simulink model "DYNctl_ver4_etud_obfusc"  (R2014b)
settings: Solver=ode45  StartTime=0.0  StopTime=tfin  FixedStep=0.001  RelTol=1e-09
values from neighbouring files (symbols this model uses):
  ae1 = 1.3463    [MatlabProjet.m]    (also in bancessai_ini.m)
  ae2 = 349.0774    [MatlabProjet.m]    (also in bancessai_ini.m)
  ae3 = 1450.3848    [MatlabProjet.m]    (also in bancessai_ini.m)
  ae4 = 703344.2113    [MatlabProjet.m]    (also in bancessai_ini.m)
  as1 = 0.052961    [MatlabProjet.m]    (also in bancessai_ini.m = -0.22862)
  as2 = 30.5716    [MatlabProjet.m]    (also in bancessai_ini.m = 176.4976)
  as3 = -1152.4168    [MatlabProjet.m]    (also in bancessai_ini.m = -16589.0203)
  as4 = 344545.4587    [MatlabProjet.m]    (also in bancessai_ini.m = 767085.5302)
  b_E1 = 13.029359254409743    (= 13.0293592544)    [MatlabProjet.m]    (also in bancEssaiConstantes.m; bancessai_ini.m; matrices_syms.m)
  g = 9.81    [MatlabProjet.m]    (also in bancEssaiConstantes.m; bancessai_ini.m; matrices_syms.m; trajectoire.m = sqrt(1 + dy.^2))
  Ixy = 0.0011691    [MatlabProjet.m]    (also in bancEssaiConstantes.m = 0.011691; bancessai_ini.m; matrices_syms.m)
  L_bobine = 115/1000    (= 0.115)    [MatlabProjet.m]    (also in bancEssaiConstantes.m; bancessai_ini.m = 115; matrices_syms.m)
  m_ps = m_plaque + m_sphere    (= 0.433)    [MatlabProjet.m]    (also in bancessai_ini.m; matrices_syms.m)
  m_sphere = 0.008    [MatlabProjet.m]    (also in bancessai_ini.m; matrices_syms.m)
  r_ABC = 95.2 / 1000    (= 0.0952)    [MatlabProjet.m]    (also in bancessai_ini.m; matrices_syms.m)
  R_bobine = 3.6    [MatlabProjet.m]    (also in bancEssaiConstantes.m; bancessai_ini.m; matrices_syms.m)
  XA = r_ABC    (= 0.0952)    [MatlabProjet.m]    (also in bancEssaiConstantes.m; bancessai_ini.m; matrices_syms.m)
  XB = -r_ABC*sind(30)    [MatlabProjet.m]    (also in bancEssaiConstantes.m = -rABC*sind(30); bancessai_ini.m; matrices_syms.m)
  XC = XB    [MatlabProjet.m]    (also in bancEssaiConstantes.m = -rABC*sind(30); bancessai_ini.m; matrices_syms.m)
  XD = r_DEF*sind(30)    [MatlabProjet.m]    (also in bancEssaiConstantes.m = +rDEF*sind(30); bancessai_ini.m; matrices_syms.m)
  XE = -r_DEF    (= -0.08)    [MatlabProjet.m]    (also in bancEssaiConstantes.m; bancessai_ini.m; matrices_syms.m)
  XF = XD    [MatlabProjet.m]    (also in bancEssaiConstantes.m = +rDEF*sind(30); bancessai_ini.m; matrices_syms.m)
  YA = 0    [MatlabProjet.m]    (also in bancEssaiConstantes.m; bancessai_ini.m; matrices_syms.m)
  YB = r_ABC*cosd(30)    [MatlabProjet.m]    (also in bancEssaiConstantes.m = +rABC*cosd(30); bancessai_ini.m; matrices_syms.m)
  YC = -YB    [MatlabProjet.m]    (also in bancEssaiConstantes.m = -rABC*cosd(30); bancessai_ini.m; matrices_syms.m)
  YD = r_DEF*cosd(30)    [MatlabProjet.m]    (also in bancEssaiConstantes.m = +rDEF*cosd(30); bancessai_ini.m; matrices_syms.m)
  YE = 0    [MatlabProjet.m]    (also in bancEssaiConstantes.m; bancessai_ini.m; matrices_syms.m)
  YF = -YD    [MatlabProjet.m]    (also in bancEssaiConstantes.m = -rDEF*cosd(30); bancessai_ini.m; matrices_syms.m)
settings Model: Creator=delafontaine  LastModifiedBy=lemg2013
settings SolverCC: AlgebraicLoopSolver=LineSearch
settings DataIOCC: SignalLoggingSaveFormat=ModelDataLogs
settings DebuggingCC: UnderspecifiedInitializationDetection=Classic  MergeDetectMultiDrivingBlocksExec=none  SolverPrmCheckMsg=none  MultiTaskDSMMsg=warning  MultiTaskCondExecSysMsg=none  FrameProcessingCompatibilityMsg=error
settings RTWCC: IncludeERTFirstTime=on

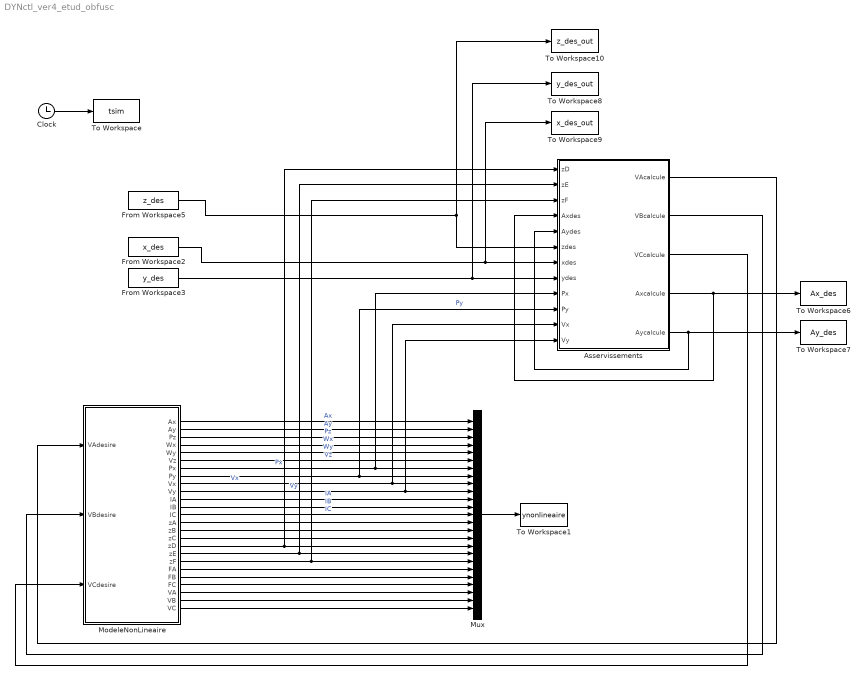
== system DYNctl_ver4_etud_obfusc ==
  Asservissements : Subsystem
      mask help: Simulink:masks:GenSFuncDesc_MD
      mask Help: eval('feval(''rtwprivate'',''rtwhelpview'',''rtw_sfcn_block'')');
  Clock : Clock
  From Workspace2 : FromWorkspace  VariableName=x_des  SampleTime=0  Interpolate=off  OutputAfterFinalValue=Holding final value
  From Workspace3 : FromWorkspace  VariableName=y_des  SampleTime=0  Interpolate=off  OutputAfterFinalValue=Holding final value
  From Workspace5 : FromWorkspace  VariableName=z_des  SampleTime=0  Interpolate=off  OutputAfterFinalValue=Holding final value
  ModeleNonLineaire : Subsystem
      mask help: Simulink:masks:GenSFuncDesc_MD
      mask Help: eval('feval(''rtwprivate'',''rtwhelpview'',''rtw_sfcn_block'')');
  Mux : Mux  Inputs=25
  To Workspace : ToWorkspace  VariableName=tsim  SampleTime=-1
  To Workspace1 : ToWorkspace  VariableName=ynonlineaire  SampleTime=-1
  To Workspace10 : ToWorkspace  VariableName=z_des_out  SampleTime=-1
  To Workspace6 : ToWorkspace  VariableName=Ax_des  SampleTime=-1
  To Workspace7 : ToWorkspace  VariableName=Ay_des  SampleTime=-1
  To Workspace8 : ToWorkspace  VariableName=y_des_out  SampleTime=-1
  To Workspace9 : ToWorkspace  VariableName=x_des_out  SampleTime=-1
  wires:
  Mux/1 -> To Workspace1/1
  Clock/1 -> To Workspace/1
  From Workspace5/1 -> Asservissements/6(zdes), To Workspace10/1
  ModeleNonLineaire/1(Ax) -> Mux/1  "Ax"
  ModeleNonLineaire/2(Ay) -> Mux/2  "Ay"
  ModeleNonLineaire/3(Pz) -> Mux/3  "Pz"
  ModeleNonLineaire/4(Wx) -> Mux/4  "Wx"
  ModeleNonLineaire/5(Wy) -> Mux/5  "Wy"
  ModeleNonLineaire/6(Vz) -> Mux/6  "Vz"
  ModeleNonLineaire/7(Px) -> Asservissements/9(Px), Mux/7  "Px"
  ModeleNonLineaire/8(Py) -> Asservissements/10(Py), Mux/8  "Py"
  ModeleNonLineaire/9(Vx) -> Asservissements/11(Vx), Mux/9  "Vx"
  ModeleNonLineaire/10(Vy) -> Asservissements/12(Vy), Mux/10  "Vy"
  ModeleNonLineaire/11(IA) -> Mux/11  "IA"
  ModeleNonLineaire/12(IB) -> Mux/12  "IB"
  ModeleNonLineaire/13(IC) -> Mux/13  "IC"
  From Workspace3/1 -> Asservissements/8(ydes), To Workspace8/1
  From Workspace2/1 -> Asservissements/7(xdes), To Workspace9/1
  ModeleNonLineaire/20(FA) -> Mux/20
  ModeleNonLineaire/21(FB) -> Mux/21
  ModeleNonLineaire/22(FC) -> Mux/22
  ModeleNonLineaire/23(VA) -> Mux/23
  ModeleNonLineaire/24(VB) -> Mux/24
  ModeleNonLineaire/25(VC) -> Mux/25
  ModeleNonLineaire/17(zD) -> Asservissements/1(zD), Mux/17
  ModeleNonLineaire/18(zE) -> Asservissements/2(zE), Mux/18
  ModeleNonLineaire/19(zF) -> Asservissements/3(zF), Mux/19
  ModeleNonLineaire/14(zA) -> Mux/14
  ModeleNonLineaire/15(zB) -> Mux/15
  ModeleNonLineaire/16(zC) -> Mux/16
  Asservissements/4(Axcalcule) -> Asservissements/4(Axdes), To Workspace6/1
  Asservissements/5(Aycalcule) -> Asservissements/5(Aydes), To Workspace7/1
  Asservissements/1(VAcalcule) -> ModeleNonLineaire/1(VAdesire)
  Asservissements/2(VBcalcule) -> ModeleNonLineaire/2(VBdesire)
  Asservissements/3(VCcalcule) -> ModeleNonLineaire/3(VCdesire)

== system DYNctl_ver4_etud_obfusc/Asservissements ==
  zD : Inport
  zE : Inport  Port=2
  zF : Inport  Port=3
  Axdes : Inport  Port=4
  Aydes : Inport  Port=5
  zdes : Inport  Port=6
  xdes : Inport  Port=7
  ydes : Inport  Port=8
  Px : Inport  Port=9
  Py : Inport  Port=10
  Vx : Inport  Port=11
  Vy : Inport  Port=12
  Asservissements_sfcn : S-Function  FunctionName=Asservissements_sf  SFunctionModules=""  EnableBusSupport=off  mask{rtw_sf_name=Asservissements_sf, showVar=off}
      mask prompts: rtw_sf_name "Simulink:masks:GenSFuncName_MP"; showVar "Simulink:masks:GenSFuncShowModuleList_MP"
      mask help: Simulink:masks:GenSFuncDesc_MD
      mask init:
      | displist = '';
      | if ~strcmp(get_param(gcb, 'FunctionName'), rtw_sf_name);
      |   set_param(gcb, 'FunctionName', rtw_sf_name);
      | end
      | % Check if we are generating code
      | rtw_mode = false;
      | if strcmpi(get_param(bdroot(gcb),'SimulationStatus'),'Initializing')
      | 	rtw_mode = strcmpi(get_param(bdroot(gcb),'BuildingRTWCode'),'on') && ...
      | 		~strcmpi(get_param(bdroot(gcb),'TargetStyle'),'SimulationTarget');
      | end
      | if showVar || rtw_mode
      | 	if exist('rtwsfunc') == 2 | exist('rtwsfunc') == 6
      | 		tmplist = rtwsfunc(rtw_sf_name,gcb);
      | 		tmplist = DAStudio.message('Simulink:masks:GenSFuncListOfModules_IC', tmplist);
      | 	elseif showVar
      | 		tmplist1 = DAStudio.message('Simulink:masks:GenSFuncListOfModules_IC', '');
      |         tmplist2 = DAStudio.message('Simulink:masks:GenSFuncNotLicensed_IC');
      |         tmplist = [tmplist1 tmplist2];
      |  	end
      | end
      | if showVar
      |   displist = tmplist;
      | end
      settings: CopyFcn=|
      | if ~strcmp(get_param(gcb,'Linkstatus'),'none') && ...
      | ~strcmp(get_param(gcb,'Linkstatus'),'implicit')
      |   set_param(gcb,'LinkStatus','none');
      | end
      mask Help: eval('feval(''rtwprivate'',''rtwhelpview'',''rtw_sfcn_block'')');
      mask Display:
      | port_label('input',1,'zD');
      | port_label('input',2,'zE');
      | port_label('input',3,'zF');
      | port_label('input',4,'Axdes');
      | port_label('input',5,'Aydes');
      | port_label('input',6,'zdes');
      | port_label('input',7,'xdes');
      | port_label('input',8,'ydes');
      | port_label('input',9,'Px');
      | port_label('input',10,'Py');
      | port_label('input',11,'Vx');
      | port_label('input',12,'Vy');
      | port_label('output',1,'VAcalcule');
      | port_label('output',2,'VBcalcule');
      | port_label('output',3,'VCcalcule');
      | port_label('output',4,'Axcalcule');
      | port_label('output',5,'Aycalcule');
  __InputSSForSFun__ : Subsystem
  __OutputSSForSFun__ : Subsystem
  VAcalcule : Outport
  VBcalcule : Outport  Port=2
  VCcalcule : Outport  Port=3
  Axcalcule : Outport  Port=4
  Aycalcule : Outport  Port=5
  wires:
  zD/1 -> __InputSSForSFun__/1(zD)
  zE/1 -> __InputSSForSFun__/2(zE)
  zF/1 -> __InputSSForSFun__/3(zF)
  Axdes/1 -> __InputSSForSFun__/4(Axdes)
  Aydes/1 -> __InputSSForSFun__/5(Aydes)
  zdes/1 -> __InputSSForSFun__/6(zdes)
  xdes/1 -> __InputSSForSFun__/7(xdes)
  ydes/1 -> __InputSSForSFun__/8(ydes)
  Px/1 -> __InputSSForSFun__/9(Px)
  Py/1 -> __InputSSForSFun__/10(Py)
  Vx/1 -> __InputSSForSFun__/11(Vx)
  Vy/1 -> __InputSSForSFun__/12(Vy)
  __InputSSForSFun__/1(__UniqueOutportName__1__) -> Asservissements_sfcn/1
  __InputSSForSFun__/2(__UniqueOutportName__2__) -> Asservissements_sfcn/2
  __InputSSForSFun__/3(__UniqueOutportName__3__) -> Asservissements_sfcn/3
  __InputSSForSFun__/4(__UniqueOutportName__4__) -> Asservissements_sfcn/4
  __InputSSForSFun__/5(__UniqueOutportName__5__) -> Asservissements_sfcn/5
  __InputSSForSFun__/6(__UniqueOutportName__6__) -> Asservissements_sfcn/6
  __InputSSForSFun__/7(__UniqueOutportName__7__) -> Asservissements_sfcn/7
  __InputSSForSFun__/8(__UniqueOutportName__8__) -> Asservissements_sfcn/8
  __InputSSForSFun__/9(__UniqueOutportName__9__) -> Asservissements_sfcn/9
  __InputSSForSFun__/10(__UniqueOutportName__10__) -> Asservissements_sfcn/10
  __InputSSForSFun__/11(__UniqueOutportName__11__) -> Asservissements_sfcn/11
  __InputSSForSFun__/12(__UniqueOutportName__12__) -> Asservissements_sfcn/12
  Asservissements_sfcn/1 -> __OutputSSForSFun__/1(__UniqueInportName__1__)
  Asservissements_sfcn/2 -> __OutputSSForSFun__/2(__UniqueInportName__2__)
  Asservissements_sfcn/3 -> __OutputSSForSFun__/3(__UniqueInportName__3__)
  Asservissements_sfcn/4 -> __OutputSSForSFun__/4(__UniqueInportName__4__)
  Asservissements_sfcn/5 -> __OutputSSForSFun__/5(__UniqueInportName__5__)
  __OutputSSForSFun__/1(VAcalcule) -> VAcalcule/1
  __OutputSSForSFun__/2(VBcalcule) -> VBcalcule/1
  __OutputSSForSFun__/3(VCcalcule) -> VCcalcule/1
  __OutputSSForSFun__/4(Axcalcule) -> Axcalcule/1
  __OutputSSForSFun__/5(Aycalcule) -> Aycalcule/1

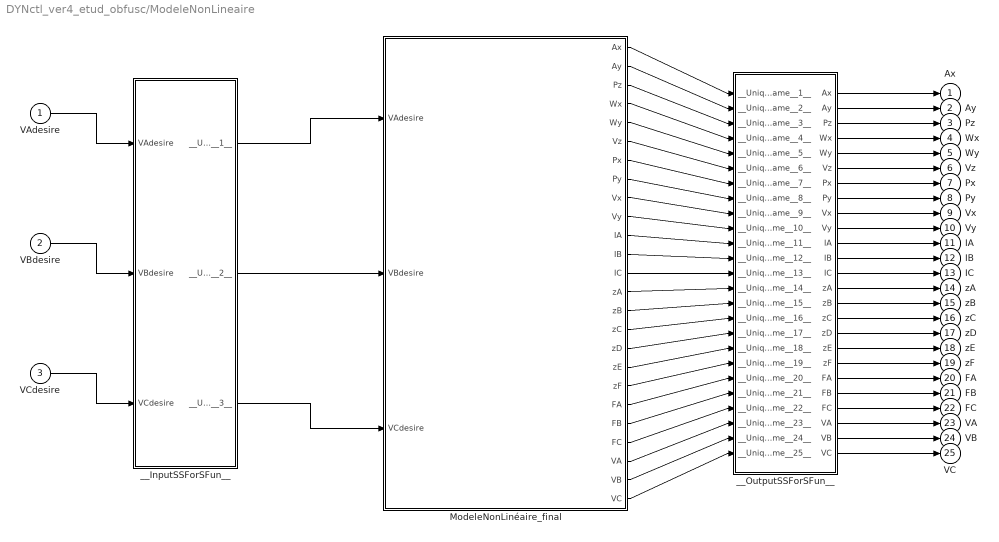
== system DYNctl_ver4_etud_obfusc/ModeleNonLineaire ==
  VAdesire : Inport
  VBdesire : Inport  Port=2
  VCdesire : Inport  Port=3
  ModeleNonLinéaire_final : Subsystem
  __InputSSForSFun__ : Subsystem
  __OutputSSForSFun__ : Subsystem
  Ax : Outport
  Ay : Outport  Port=2
  Pz : Outport  Port=3
  Wx : Outport  Port=4
  Wy : Outport  Port=5
  Vz : Outport  Port=6
  Px : Outport  Port=7
  Py : Outport  Port=8
  Vx : Outport  Port=9
  Vy : Outport  Port=10
  IA : Outport  Port=11
  IB : Outport  Port=12
  IC : Outport  Port=13
  zA : Outport  Port=14
  zB : Outport  Port=15
  zC : Outport  Port=16
  zD : Outport  Port=17
  zE : Outport  Port=18
  zF : Outport  Port=19
  FA : Outport  Port=20
  FB : Outport  Port=21
  FC : Outport  Port=22
  VA : Outport  Port=23
  VB : Outport  Port=24
  VC : Outport  Port=25
  wires:
  VAdesire/1 -> __InputSSForSFun__/1(VAdesire)
  VBdesire/1 -> __InputSSForSFun__/2(VBdesire)
  VCdesire/1 -> __InputSSForSFun__/3(VCdesire)
  __InputSSForSFun__/1(__UniqueOutportName__1__) -> ModeleNonLinéaire_final/1(VAdesire)
  ModeleNonLinéaire_final/1(Ax) -> __OutputSSForSFun__/1(__UniqueInportName__1__)
  ModeleNonLinéaire_final/2(Ay) -> __OutputSSForSFun__/2(__UniqueInportName__2__)
  ModeleNonLinéaire_final/3(Pz) -> __OutputSSForSFun__/3(__UniqueInportName__3__)
  ModeleNonLinéaire_final/4(Wx) -> __OutputSSForSFun__/4(__UniqueInportName__4__)
  ModeleNonLinéaire_final/5(Wy) -> __OutputSSForSFun__/5(__UniqueInportName__5__)
  ModeleNonLinéaire_final/6(Vz) -> __OutputSSForSFun__/6(__UniqueInportName__6__)
  ModeleNonLinéaire_final/7(Px) -> __OutputSSForSFun__/7(__UniqueInportName__7__)
  ModeleNonLinéaire_final/8(Py) -> __OutputSSForSFun__/8(__UniqueInportName__8__)
  ModeleNonLinéaire_final/9(Vx) -> __OutputSSForSFun__/9(__UniqueInportName__9__)
  ModeleNonLinéaire_final/10(Vy) -> __OutputSSForSFun__/10(__UniqueInportName__10__)
  ModeleNonLinéaire_final/11(IA) -> __OutputSSForSFun__/11(__UniqueInportName__11__)
  ModeleNonLinéaire_final/12(IB) -> __OutputSSForSFun__/12(__UniqueInportName__12__)
  ModeleNonLinéaire_final/13(IC) -> __OutputSSForSFun__/13(__UniqueInportName__13__)
  ModeleNonLinéaire_final/14(zA) -> __OutputSSForSFun__/14(__UniqueInportName__14__)
  ModeleNonLinéaire_final/15(zB) -> __OutputSSForSFun__/15(__UniqueInportName__15__)
  ModeleNonLinéaire_final/16(zC) -> __OutputSSForSFun__/16(__UniqueInportName__16__)
  ModeleNonLinéaire_final/17(zD) -> __OutputSSForSFun__/17(__UniqueInportName__17__)
  ModeleNonLinéaire_final/18(zE) -> __OutputSSForSFun__/18(__UniqueInportName__18__)
  ModeleNonLinéaire_final/19(zF) -> __OutputSSForSFun__/19(__UniqueInportName__19__)
  ModeleNonLinéaire_final/20(FA) -> __OutputSSForSFun__/20(__UniqueInportName__20__)
  ModeleNonLinéaire_final/21(FB) -> __OutputSSForSFun__/21(__UniqueInportName__21__)
  ModeleNonLinéaire_final/22(FC) -> __OutputSSForSFun__/22(__UniqueInportName__22__)
  ModeleNonLinéaire_final/23(VA) -> __OutputSSForSFun__/23(__UniqueInportName__23__)
  ModeleNonLinéaire_final/24(VB) -> __OutputSSForSFun__/24(__UniqueInportName__24__)
  ModeleNonLinéaire_final/25(VC) -> __OutputSSForSFun__/25(__UniqueInportName__25__)
  __OutputSSForSFun__/1(Ax) -> Ax/1
  __OutputSSForSFun__/2(Ay) -> Ay/1
  __OutputSSForSFun__/3(Pz) -> Pz/1
  __OutputSSForSFun__/4(Wx) -> Wx/1
  __OutputSSForSFun__/5(Wy) -> Wy/1
  __OutputSSForSFun__/6(Vz) -> Vz/1
  __OutputSSForSFun__/7(Px) -> Px/1
  __OutputSSForSFun__/8(Py) -> Py/1
  __OutputSSForSFun__/9(Vx) -> Vx/1
  __OutputSSForSFun__/10(Vy) -> Vy/1
  __OutputSSForSFun__/11(IA) -> IA/1
  __OutputSSForSFun__/12(IB) -> IB/1
  __OutputSSForSFun__/13(IC) -> IC/1
  __OutputSSForSFun__/14(zA) -> zA/1
  __OutputSSForSFun__/15(zB) -> zB/1
  __OutputSSForSFun__/16(zC) -> zC/1
  __OutputSSForSFun__/17(zD) -> zD/1
  __OutputSSForSFun__/18(zE) -> zE/1
  __OutputSSForSFun__/19(zF) -> zF/1
  __OutputSSForSFun__/20(FA) -> FA/1
  __OutputSSForSFun__/21(FB) -> FB/1
  __OutputSSForSFun__/22(FC) -> FC/1
  __OutputSSForSFun__/23(VA) -> VA/1
  __OutputSSForSFun__/24(VB) -> VB/1
  __OutputSSForSFun__/25(VC) -> VC/1
  __InputSSForSFun__/2(__UniqueOutportName__2__) -> ModeleNonLinéaire_final/2(VBdesire)
  __InputSSForSFun__/3(__UniqueOutportName__3__) -> ModeleNonLinéaire_final/3(VCdesire)

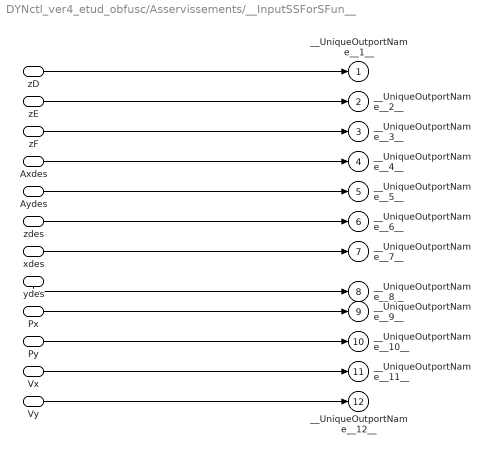
== system DYNctl_ver4_etud_obfusc/Asservissements/__InputSSForSFun__ ==
  zD : Inport
  zE : Inport  Port=2
  zF : Inport  Port=3
  Axdes : Inport  Port=4
  Aydes : Inport  Port=5
  zdes : Inport  Port=6
  xdes : Inport  Port=7
  ydes : Inport  Port=8
  Px : Inport  Port=9
  Py : Inport  Port=10
  Vx : Inport  Port=11
  Vy : Inport  Port=12
  __UniqueOutportName__1__ : Outport
  __UniqueOutportName__2__ : Outport  Port=2
  __UniqueOutportName__3__ : Outport  Port=3
  __UniqueOutportName__4__ : Outport  Port=4
  __UniqueOutportName__5__ : Outport  Port=5
  __UniqueOutportName__6__ : Outport  Port=6
  __UniqueOutportName__7__ : Outport  Port=7
  __UniqueOutportName__8__ : Outport  Port=8
  __UniqueOutportName__9__ : Outport  Port=9
  __UniqueOutportName__10__ : Outport  Port=10
  __UniqueOutportName__11__ : Outport  Port=11
  __UniqueOutportName__12__ : Outport  Port=12
  wires:
  zD/1 -> __UniqueOutportName__1__/1
  zE/1 -> __UniqueOutportName__2__/1
  zF/1 -> __UniqueOutportName__3__/1
  Axdes/1 -> __UniqueOutportName__4__/1
  Aydes/1 -> __UniqueOutportName__5__/1
  zdes/1 -> __UniqueOutportName__6__/1
  xdes/1 -> __UniqueOutportName__7__/1
  ydes/1 -> __UniqueOutportName__8__/1
  Px/1 -> __UniqueOutportName__9__/1
  Py/1 -> __UniqueOutportName__10__/1
  Vx/1 -> __UniqueOutportName__11__/1
  Vy/1 -> __UniqueOutportName__12__/1

== system DYNctl_ver4_etud_obfusc/Asservissements/__OutputSSForSFun__ ==
  __UniqueInportName__1__ : Inport
  __UniqueInportName__2__ : Inport  Port=2
  __UniqueInportName__3__ : Inport  Port=3
  __UniqueInportName__4__ : Inport  Port=4
  __UniqueInportName__5__ : Inport  Port=5
  VAcalcule : Outport
  VBcalcule : Outport  Port=2
  VCcalcule : Outport  Port=3
  Axcalcule : Outport  Port=4
  Aycalcule : Outport  Port=5
  wires:
  __UniqueInportName__1__/1 -> VAcalcule/1
  __UniqueInportName__2__/1 -> VBcalcule/1
  __UniqueInportName__3__/1 -> VCcalcule/1
  __UniqueInportName__4__/1 -> Axcalcule/1  "Ax_des"
  __UniqueInportName__5__/1 -> Aycalcule/1  "Ay_des"

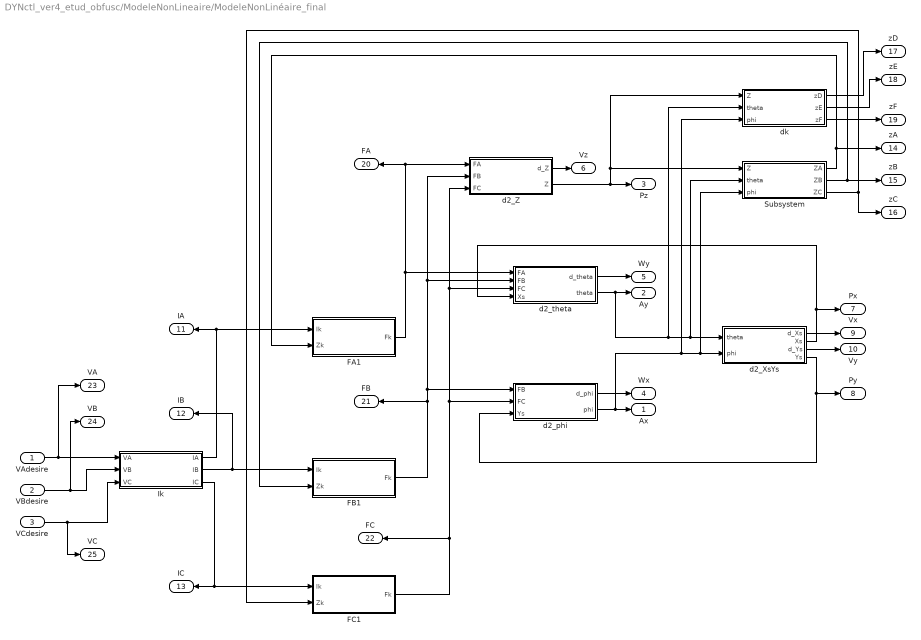
== system DYNctl_ver4_etud_obfusc/ModeleNonLineaire/ModeleNonLinéaire_final ==
  VAdesire : Inport
  VBdesire : Inport  Port=2
  VCdesire : Inport  Port=3
  FA1 : Subsystem
  FB1 : Subsystem
  FC1 : Subsystem
  Ik : Subsystem
  Subsystem : Subsystem
  d2_XsYs : Subsystem
  d2_Z : Subsystem
  d2_phi : Subsystem
  d2_theta : Subsystem
  dk : Subsystem
  Ax : Outport
  Ay : Outport  Port=2
  Pz : Outport  Port=3
  Wx : Outport  Port=4
  Wy : Outport  Port=5
  Vz : Outport  Port=6
  Px : Outport  Port=7
  Py : Outport  Port=8
  Vx : Outport  Port=9
  Vy : Outport  Port=10
  IA : Outport  Port=11
  IB : Outport  Port=12
  IC : Outport  Port=13
  zA : Outport  Port=14
  zB : Outport  Port=15
  zC : Outport  Port=16
  zD : Outport  Port=17
  zE : Outport  Port=18
  zF : Outport  Port=19
  FA : Outport  Port=20
  FB : Outport  Port=21
  FC : Outport  Port=22
  VA : Outport  Port=23
  VB : Outport  Port=24
  VC : Outport  Port=25
  wires:
  VAdesire/1 -> VA/1, Ik/1(VA)
  VBdesire/1 -> VB/1, Ik/2(VB)
  VCdesire/1 -> VC/1, Ik/3(VC)
  Ik/1(IA) -> IA/1, FA1/1(Ik)
  Ik/2(IB) -> IB/1, FB1/1(Ik)
  Ik/3(IC) -> IC/1, FC1/1(Ik)
  FA1/1(Fk) -> d2_theta/1(FA), FA/1, d2_Z/1(FA)
  FB1/1(Fk) -> d2_phi/1(FB), d2_theta/2(FB), d2_Z/2(FB), FB/1
  FC1/1(Fk) -> FC/1, d2_phi/2(FC), d2_theta/3(FC), d2_Z/3(FC)
  d2_phi/2("phi ") -> Ax/1, dk/3(phi), Subsystem/3(phi), d2_XsYs/2(phi)
  d2_theta/2("theta ") -> Ay/1, dk/2(theta), Subsystem/2(theta), d2_XsYs/1(theta)
  d2_XsYs/2(Xs) -> Px/1, d2_theta/4(Xs)
  d2_XsYs/4(Ys) -> Py/1, d2_phi/3(Ys)
  d2_Z/2(Z) -> Pz/1, dk/1(Z), Subsystem/1(Z)
  Subsystem/1(ZA) -> zA/1, FA1/2(Zk)
  Subsystem/2(ZB) -> zB/1, FB1/2(Zk)
  Subsystem/3(ZC) -> zC/1, FC1/2(Zk)
  d2_phi/1("d_phi ") -> Wx/1
  d2_theta/1("d_theta ") -> Wy/1
  d2_Z/1(d_Z) -> Vz/1
  d2_XsYs/1(d_Xs) -> Vx/1
  d2_XsYs/3(d_Ys) -> Vy/1
  dk/1(zD) -> zD/1
  dk/2(zE) -> zE/1
  dk/3(zF) -> zF/1

== system DYNctl_ver4_etud_obfusc/ModeleNonLineaire/__InputSSForSFun__ ==
  VAdesire : Inport
  VBdesire : Inport  Port=2
  VCdesire : Inport  Port=3
  __UniqueOutportName__1__ : Outport
  __UniqueOutportName__2__ : Outport  Port=2
  __UniqueOutportName__3__ : Outport  Port=3
  wires:
  VAdesire/1 -> __UniqueOutportName__1__/1
  VBdesire/1 -> __UniqueOutportName__2__/1
  VCdesire/1 -> __UniqueOutportName__3__/1

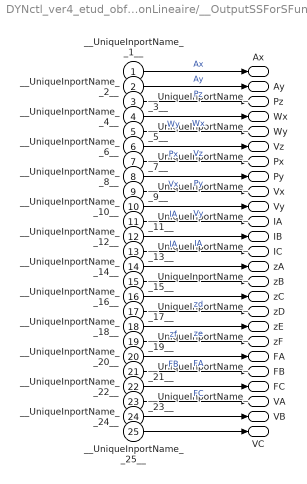
== system DYNctl_ver4_etud_obfusc/ModeleNonLineaire/__OutputSSForSFun__ ==
  __UniqueInportName__1__ : Inport
  __UniqueInportName__2__ : Inport  Port=2
  __UniqueInportName__3__ : Inport  Port=3
  __UniqueInportName__4__ : Inport  Port=4
  __UniqueInportName__5__ : Inport  Port=5
  __UniqueInportName__6__ : Inport  Port=6
  __UniqueInportName__7__ : Inport  Port=7
  __UniqueInportName__8__ : Inport  Port=8
  __UniqueInportName__9__ : Inport  Port=9
  __UniqueInportName__10__ : Inport  Port=10
  __UniqueInportName__11__ : Inport  Port=11
  __UniqueInportName__12__ : Inport  Port=12
  __UniqueInportName__13__ : Inport  Port=13
  __UniqueInportName__14__ : Inport  Port=14
  __UniqueInportName__15__ : Inport  Port=15
  __UniqueInportName__16__ : Inport  Port=16
  __UniqueInportName__17__ : Inport  Port=17
  __UniqueInportName__18__ : Inport  Port=18
  __UniqueInportName__19__ : Inport  Port=19
  __UniqueInportName__20__ : Inport  Port=20
  __UniqueInportName__21__ : Inport  Port=21
  __UniqueInportName__22__ : Inport  Port=22
  __UniqueInportName__23__ : Inport  Port=23
  __UniqueInportName__24__ : Inport  Port=24
  __UniqueInportName__25__ : Inport  Port=25
  Ax : Outport
  Ay : Outport  Port=2
  Pz : Outport  Port=3
  Wx : Outport  Port=4
  Wy : Outport  Port=5
  Vz : Outport  Port=6
  Px : Outport  Port=7
  Py : Outport  Port=8
  Vx : Outport  Port=9
  Vy : Outport  Port=10
  IA : Outport  Port=11
  IB : Outport  Port=12
  IC : Outport  Port=13
  zA : Outport  Port=14
  zB : Outport  Port=15
  zC : Outport  Port=16
  zD : Outport  Port=17
  zE : Outport  Port=18
  zF : Outport  Port=19
  FA : Outport  Port=20
  FB : Outport  Port=21
  FC : Outport  Port=22
  VA : Outport  Port=23
  VB : Outport  Port=24
  VC : Outport  Port=25
  wires:
  __UniqueInportName__1__/1 -> Ax/1  "Ax"
  __UniqueInportName__2__/1 -> Ay/1  "Ay"
  __UniqueInportName__3__/1 -> Pz/1  "Pz"
  __UniqueInportName__4__/1 -> Wx/1  "Wx"
  __UniqueInportName__5__/1 -> Wy/1  "Wy"
  __UniqueInportName__6__/1 -> Vz/1  "Vz"
  __UniqueInportName__7__/1 -> Px/1  "Px"
  __UniqueInportName__8__/1 -> Py/1  "Py"
  __UniqueInportName__9__/1 -> Vx/1  "Vx"
  __UniqueInportName__10__/1 -> Vy/1  "Vy"
  __UniqueInportName__11__/1 -> IA/1  "IA"
  __UniqueInportName__12__/1 -> IB/1  "IA"
  __UniqueInportName__13__/1 -> IC/1  "IA"
  __UniqueInportName__14__/1 -> zA/1
  __UniqueInportName__15__/1 -> zB/1
  __UniqueInportName__16__/1 -> zC/1
  __UniqueInportName__17__/1 -> zD/1  "zd"
  __UniqueInportName__18__/1 -> zE/1  "ze"
  __UniqueInportName__19__/1 -> zF/1  "zf"
  __UniqueInportName__20__/1 -> FA/1  "FA"
  __UniqueInportName__21__/1 -> FB/1  "FB"
  __UniqueInportName__22__/1 -> FC/1  "FC"
  __UniqueInportName__23__/1 -> VA/1
  __UniqueInportName__24__/1 -> VB/1
  __UniqueInportName__25__/1 -> VC/1

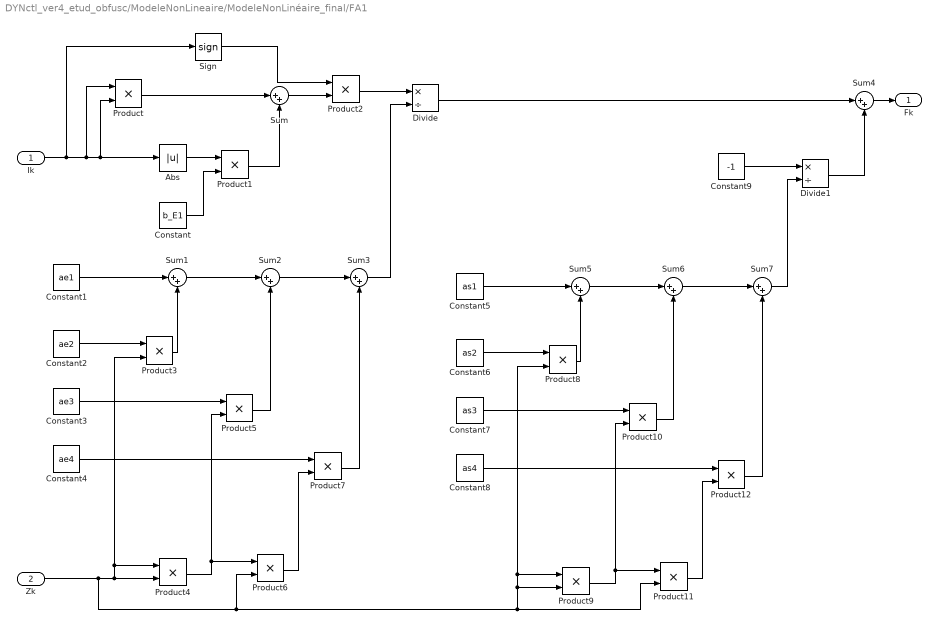
== system DYNctl_ver4_etud_obfusc/ModeleNonLineaire/ModeleNonLinéaire_final/FA1 ==
  Ik : Inport
  Zk : Inport  Port=2
  Abs : Abs
  Constant : Constant  Value=b_E1
  Constant1 : Constant  Value=ae1
  Constant2 : Constant  Value=ae2
  Constant3 : Constant  Value=ae3
  Constant4 : Constant  Value=ae4
  Constant5 : Constant  Value=as1
  Constant6 : Constant  Value=as2
  Constant7 : Constant  Value=as3
  Constant8 : Constant  Value=as4
  Constant9 : Constant  Value=-1
  Divide : Product  Inputs=*/
  Divide1 : Product  Inputs=*/
  Product{,1..12} (13 alike) : Product
  Sign : Signum
  Sum{,1..7} (8 alike) : Sum  Inputs=|++
  Fk : Outport
  wires:
  Ik/1 -> Sign/1, Product/1, Abs/1, Product/2
  Abs/1 -> Product1/1
  Constant/1 -> Product1/2
  Product1/1 -> Sum/2
  Product/1 -> Sum/1
  Sum/1 -> Product2/2
  Sign/1 -> Product2/1
  Constant1/1 -> Sum1/1
  Constant2/1 -> Product3/1
  Product3/1 -> Sum1/2
  Sum1/1 -> Sum2/1
  Product4/1 -> Product6/1, Product5/2
  Constant3/1 -> Product5/1
  Product5/1 -> Sum2/2
  Constant4/1 -> Product7/1
  Product6/1 -> Product7/2
  Product7/1 -> Sum3/2
  Sum2/1 -> Sum3/1
  Product2/1 -> Divide/1
  Sum3/1 -> Divide/2
  Constant5/1 -> Sum5/1
  Constant6/1 -> Product8/1
  Zk/1 -> Product11/2, Product8/2, Product9/1, Product9/2, Product6/2, Product3/2, Product4/1, Product4/2
  Product8/1 -> Sum5/2
  Sum5/1 -> Sum6/1
  Product9/1 -> Product11/1, Product10/2
  Constant7/1 -> Product10/1
  Product10/1 -> Sum6/2
  Constant8/1 -> Product12/1
  Product11/1 -> Product12/2
  Product12/1 -> Sum7/2
  Sum6/1 -> Sum7/1
  Sum7/1 -> Divide1/2
  Divide/1 -> Sum4/1
  Constant9/1 -> Divide1/1
  Divide1/1 -> Sum4/2
  Sum4/1 -> Fk/1

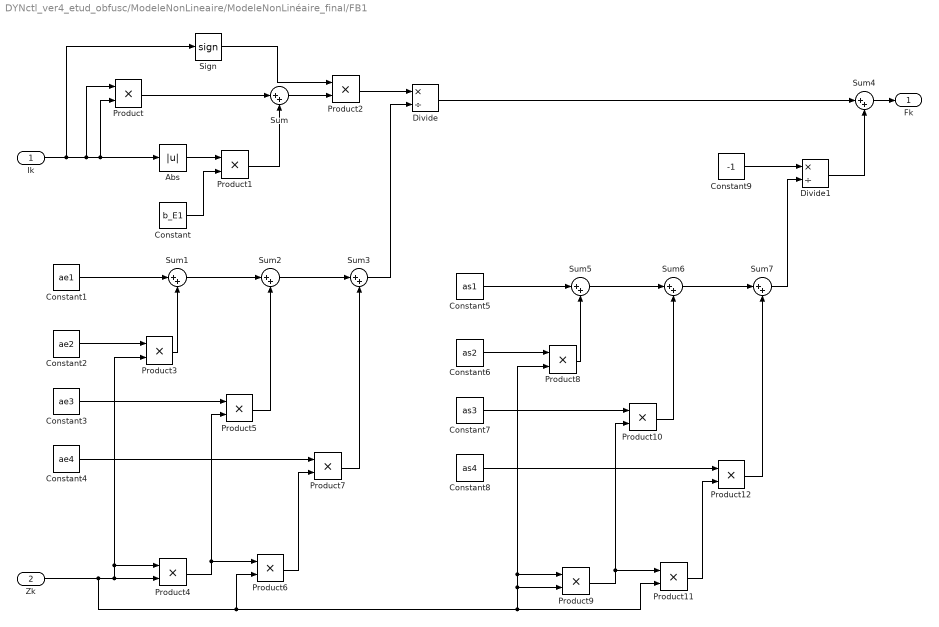
== system DYNctl_ver4_etud_obfusc/ModeleNonLineaire/ModeleNonLinéaire_final/FB1 ==
  Ik : Inport
  Zk : Inport  Port=2
  Abs : Abs
  Constant : Constant  Value=b_E1
  Constant1 : Constant  Value=ae1
  Constant2 : Constant  Value=ae2
  Constant3 : Constant  Value=ae3
  Constant4 : Constant  Value=ae4
  Constant5 : Constant  Value=as1
  Constant6 : Constant  Value=as2
  Constant7 : Constant  Value=as3
  Constant8 : Constant  Value=as4
  Constant9 : Constant  Value=-1
  Divide : Product  Inputs=*/
  Divide1 : Product  Inputs=*/
  Product{,1..12} (13 alike) : Product
  Sign : Signum
  Sum{,1..7} (8 alike) : Sum  Inputs=|++
  Fk : Outport
  wires:
  Ik/1 -> Sign/1, Product/1, Abs/1, Product/2
  Abs/1 -> Product1/1
  Constant/1 -> Product1/2
  Product1/1 -> Sum/2
  Product/1 -> Sum/1
  Sum/1 -> Product2/2
  Sign/1 -> Product2/1
  Constant1/1 -> Sum1/1
  Constant2/1 -> Product3/1
  Product3/1 -> Sum1/2
  Sum1/1 -> Sum2/1
  Product4/1 -> Product6/1, Product5/2
  Constant3/1 -> Product5/1
  Product5/1 -> Sum2/2
  Constant4/1 -> Product7/1
  Product6/1 -> Product7/2
  Product7/1 -> Sum3/2
  Sum2/1 -> Sum3/1
  Product2/1 -> Divide/1
  Sum3/1 -> Divide/2
  Constant5/1 -> Sum5/1
  Constant6/1 -> Product8/1
  Zk/1 -> Product11/2, Product8/2, Product9/1, Product9/2, Product6/2, Product3/2, Product4/1, Product4/2
  Product8/1 -> Sum5/2
  Sum5/1 -> Sum6/1
  Product9/1 -> Product11/1, Product10/2
  Constant7/1 -> Product10/1
  Product10/1 -> Sum6/2
  Constant8/1 -> Product12/1
  Product11/1 -> Product12/2
  Product12/1 -> Sum7/2
  Sum6/1 -> Sum7/1
  Sum7/1 -> Divide1/2
  Divide/1 -> Sum4/1
  Constant9/1 -> Divide1/1
  Divide1/1 -> Sum4/2
  Sum4/1 -> Fk/1

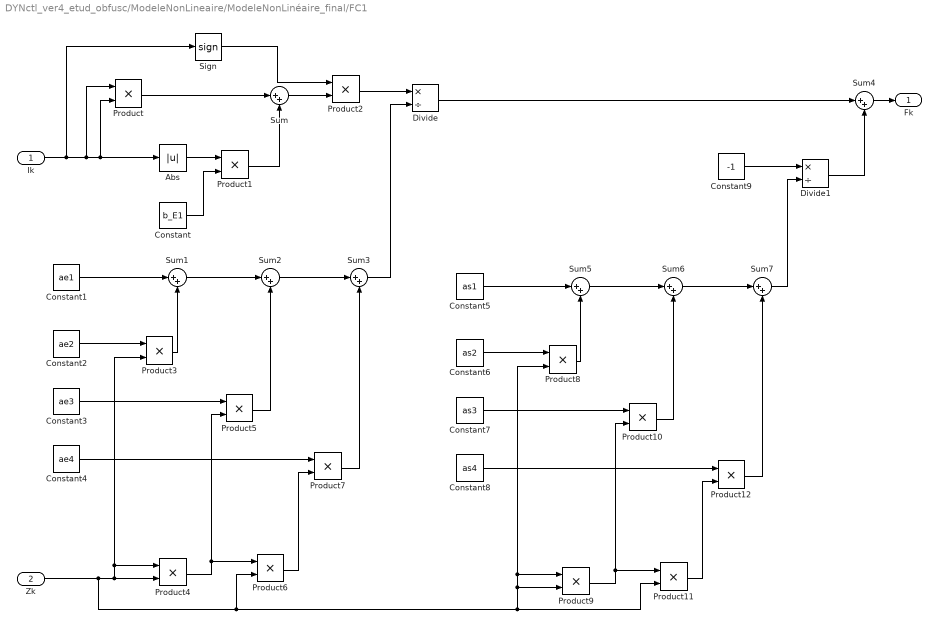
== system DYNctl_ver4_etud_obfusc/ModeleNonLineaire/ModeleNonLinéaire_final/FC1 ==
  Ik : Inport
  Zk : Inport  Port=2
  Abs : Abs
  Constant : Constant  Value=b_E1
  Constant1 : Constant  Value=ae1
  Constant2 : Constant  Value=ae2
  Constant3 : Constant  Value=ae3
  Constant4 : Constant  Value=ae4
  Constant5 : Constant  Value=as1
  Constant6 : Constant  Value=as2
  Constant7 : Constant  Value=as3
  Constant8 : Constant  Value=as4
  Constant9 : Constant  Value=-1
  Divide : Product  Inputs=*/
  Divide1 : Product  Inputs=*/
  Product{,1..12} (13 alike) : Product
  Sign : Signum
  Sum{,1..7} (8 alike) : Sum  Inputs=|++
  Fk : Outport
  wires:
  Ik/1 -> Sign/1, Product/1, Abs/1, Product/2
  Abs/1 -> Product1/1
  Constant/1 -> Product1/2
  Product1/1 -> Sum/2
  Product/1 -> Sum/1
  Sum/1 -> Product2/2
  Sign/1 -> Product2/1
  Constant1/1 -> Sum1/1
  Constant2/1 -> Product3/1
  Product3/1 -> Sum1/2
  Sum1/1 -> Sum2/1
  Product4/1 -> Product6/1, Product5/2
  Constant3/1 -> Product5/1
  Product5/1 -> Sum2/2
  Constant4/1 -> Product7/1
  Product6/1 -> Product7/2
  Product7/1 -> Sum3/2
  Sum2/1 -> Sum3/1
  Product2/1 -> Divide/1
  Sum3/1 -> Divide/2
  Constant5/1 -> Sum5/1
  Constant6/1 -> Product8/1
  Zk/1 -> Product11/2, Product8/2, Product9/1, Product9/2, Product6/2, Product3/2, Product4/1, Product4/2
  Product8/1 -> Sum5/2
  Sum5/1 -> Sum6/1
  Product9/1 -> Product11/1, Product10/2
  Constant7/1 -> Product10/1
  Product10/1 -> Sum6/2
  Constant8/1 -> Product12/1
  Product11/1 -> Product12/2
  Product12/1 -> Sum7/2
  Sum6/1 -> Sum7/1
  Sum7/1 -> Divide1/2
  Divide/1 -> Sum4/1
  Constant9/1 -> Divide1/1
  Divide1/1 -> Sum4/2
  Sum4/1 -> Fk/1

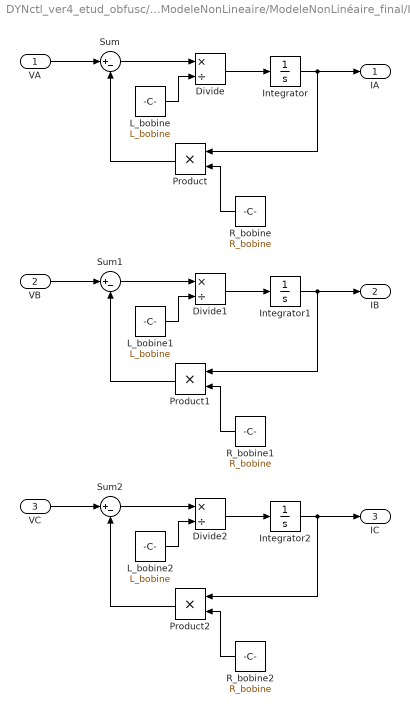
== system DYNctl_ver4_etud_obfusc/ModeleNonLineaire/ModeleNonLinéaire_final/Ik ==
  VA : Inport
  VB : Inport  Port=2
  VC : Inport  Port=3
  Divide : Product  Inputs=*/
  Divide1 : Product  Inputs=*/
  Divide2 : Product  Inputs=*/
  Integrator : Integrator
  Integrator1 : Integrator
  Integrator2 : Integrator
  L_bobine : Constant  Value=L_bobine
  L_bobine1 : Constant  Value=L_bobine
  L_bobine2 : Constant  Value=L_bobine
  Product : Product
  Product1 : Product
  Product2 : Product
  R_bobine : Constant  Value=R_bobine
  R_bobine1 : Constant  Value=R_bobine
  R_bobine2 : Constant  Value=R_bobine
  Sum : Sum  Inputs=|+-
  Sum1 : Sum  Inputs=|+-
  Sum2 : Sum  Inputs=|+-
  IA : Outport
  IB : Outport  Port=2
  IC : Outport  Port=3
  wires:
  Sum/1 -> Divide/1
  L_bobine/1 -> Divide/2
  Divide/1 -> Integrator/1
  Integrator/1 -> IA/1, Product/1
  R_bobine/1 -> Product/2
  Product/1 -> Sum/2
  VA/1 -> Sum/1
  Sum1/1 -> Divide1/1
  L_bobine1/1 -> Divide1/2
  Divide1/1 -> Integrator1/1
  Integrator1/1 -> IB/1, Product1/1
  R_bobine1/1 -> Product1/2
  Product1/1 -> Sum1/2
  VB/1 -> Sum1/1
  Sum2/1 -> Divide2/1
  L_bobine2/1 -> Divide2/2
  Divide2/1 -> Integrator2/1
  Integrator2/1 -> IC/1, Product2/1
  R_bobine2/1 -> Product2/2
  Product2/1 -> Sum2/2
  VC/1 -> Sum2/1

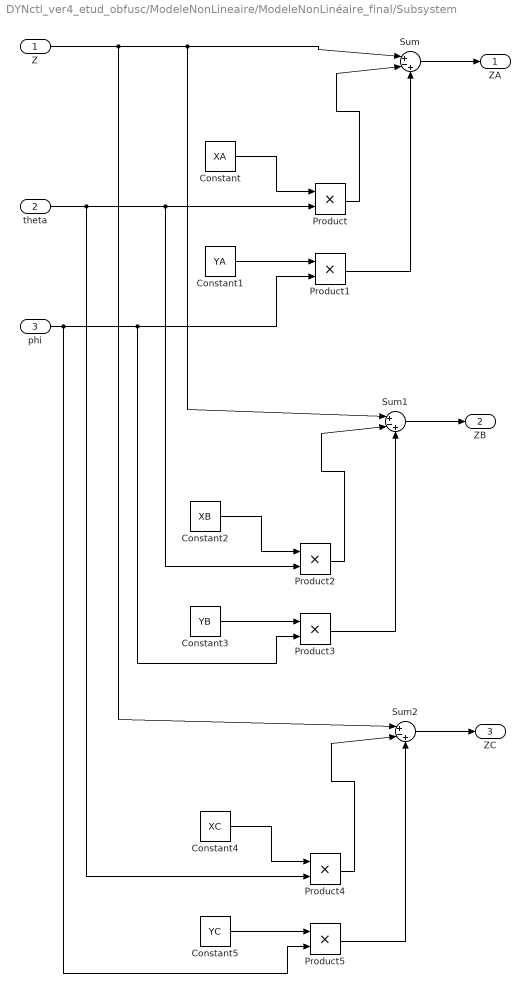
== system DYNctl_ver4_etud_obfusc/ModeleNonLineaire/ModeleNonLinéaire_final/Subsystem ==
  Z : Inport
  theta : Inport  Port=2
  phi : Inport  Port=3
  Constant : Constant  Value=XA
  Constant1 : Constant  Value=YA
  Constant2 : Constant  Value=XB
  Constant3 : Constant  Value=YB
  Constant4 : Constant  Value=XC
  Constant5 : Constant  Value=YC
  Product{,1..5} (6 alike) : Product
  Sum : Sum  Inputs=|+-+
  Sum1 : Sum  Inputs=|+-+
  Sum2 : Sum  Inputs=|+-+
  ZA : Outport
  ZB : Outport  Port=2
  ZC : Outport  Port=3
  wires:
  Constant/1 -> Product/1
  Product/1 -> Sum/2
  Constant1/1 -> Product1/1
  Product1/1 -> Sum/3
  Sum/1 -> ZA/1
  Z/1 -> Sum2/1, Sum1/1, Sum/1
  theta/1 -> Product2/2, Product/2, Product4/2
  Constant2/1 -> Product2/1
  Product2/1 -> Sum1/2
  Constant3/1 -> Product3/1
  phi/1 -> Product3/2, Product1/2, Product5/2
  Product3/1 -> Sum1/3
  Sum1/1 -> ZB/1
  Constant4/1 -> Product4/1
  Product4/1 -> Sum2/2
  Constant5/1 -> Product5/1
  Product5/1 -> Sum2/3
  Sum2/1 -> ZC/1

== system DYNctl_ver4_etud_obfusc/ModeleNonLineaire/ModeleNonLinéaire_final/d2_XsYs ==
  theta : Inport
  phi : Inport  Port=2
  Constant : Constant  Value=-g/1.4
  Constant1 : Constant  Value=g/1.4
  Integrator{,1..3} (4 alike) : Integrator
  Product : Product
  Product1 : Product
  d_Xs : Outport
  Xs : Outport  Port=2
  d_Ys : Outport  Port=3
  Ys : Outport  Port=4
  wires:
  theta/1 -> Product/1
  Constant/1 -> Product/2
  Product/1 -> Integrator/1
  Integrator/1 -> d_Xs/1, Integrator1/1
  Integrator1/1 -> Xs/1
  phi/1 -> Product1/1
  Constant1/1 -> Product1/2
  Product1/1 -> Integrator2/1
  Integrator2/1 -> d_Ys/1, Integrator3/1
  Integrator3/1 -> Ys/1

== system DYNctl_ver4_etud_obfusc/ModeleNonLineaire/ModeleNonLinéaire_final/d2_Z ==
  FA : Inport
  FB : Inport  Port=2
  FC : Inport  Port=3
  Constant : Constant  Value=m_ps
  Constant1 : Constant  Value=g
  Divide : Product  Inputs=*/
  Integrator : Integrator
  Integrator1 : Integrator
  Product : Product
  Sum : Sum  Inputs=++++
  d_Z : Outport
  Z : Outport  Port=2
  wires:
  FB/1 -> Sum/2
  FA/1 -> Sum/1
  FC/1 -> Sum/3
  Constant1/1 -> Product/2
  Product/1 -> Sum/4
  Sum/1 -> Divide/1
  Constant/1 -> Divide/2, Product/1
  Divide/1 -> Integrator/1
  Integrator1/1 -> Z/1
  Integrator/1 -> Integrator1/1, d_Z/1

== system DYNctl_ver4_etud_obfusc/ModeleNonLineaire/ModeleNonLinéaire_final/d2_phi ==
  FB : Inport
  FC : Inport  Port=2
  Ys : Inport  Port=3
  Constant : Constant  Value=Ixy
  Divide : Product  Inputs=*/
  Integrator : Integrator
  Integrator1 : Integrator
  Product{,1..4} (5 alike) : Product
  Sum : Sum  Inputs=|+-
  Sum1 : Sum  Inputs=|++
  cos30 : Constant  Value=cosd(30)
  g : Constant  Value=g
  m_sphere : Constant  Value=m_sphere
  r_ABC : Constant  Value=r_ABC
  "d_phi " : Outport
  "phi " : Outport  Port=2
  wires:
  cos30/1 -> Product/2, Product1/1
  FB/1 -> Product/1
  FC/1 -> Product1/2
  Product/1 -> Sum/1
  Product1/1 -> Sum/2
  Sum/1 -> Product2/1
  r_ABC/1 -> Product2/2
  Product2/1 -> Sum1/1
  m_sphere/1 -> Product3/1
  g/1 -> Product3/2
  Product3/1 -> Product4/2
  Ys/1 -> Product4/1
  Product4/1 -> Sum1/2
  Sum1/1 -> Divide/1
  Constant/1 -> Divide/2
  Divide/1 -> Integrator/1
  Integrator/1 -> "d_phi "/1, Integrator1/1
  Integrator1/1 -> "phi "/1

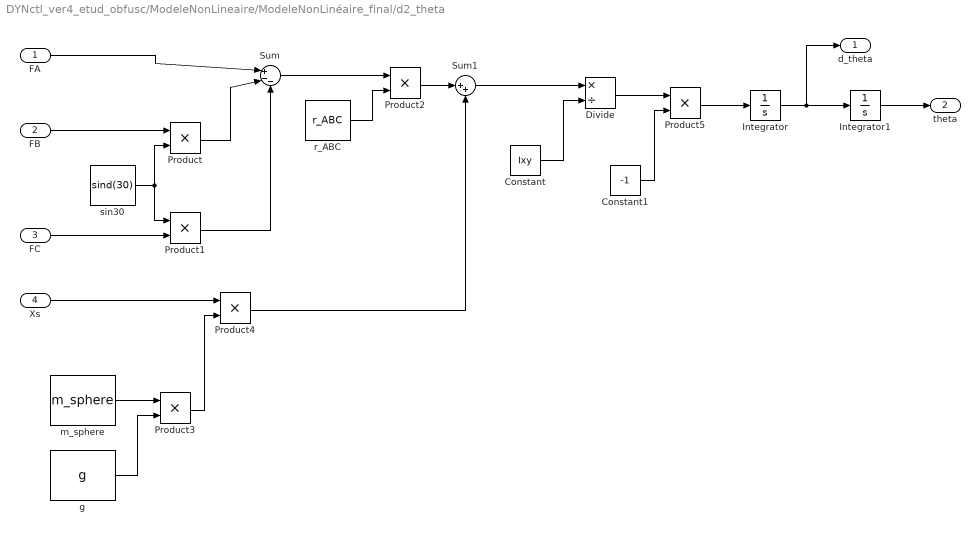
== system DYNctl_ver4_etud_obfusc/ModeleNonLineaire/ModeleNonLinéaire_final/d2_theta ==
  FA : Inport
  FB : Inport  Port=2
  FC : Inport  Port=3
  Xs : Inport  Port=4
  Constant : Constant  Value=Ixy
  Constant1 : Constant  Value=-1
  Divide : Product  Inputs=*/
  Integrator : Integrator
  Integrator1 : Integrator
  Product{,1..5} (6 alike) : Product
  Sum : Sum  Inputs=|+--
  Sum1 : Sum  Inputs=|++
  g : Constant  Value=g
  m_sphere : Constant  Value=m_sphere
  r_ABC : Constant  Value=r_ABC
  sin30 : Constant  Value=sind(30)
  "d_theta " : Outport
  "theta " : Outport  Port=2
  wires:
  sin30/1 -> Product/2, Product1/1
  FB/1 -> Product/1
  FC/1 -> Product1/2
  FA/1 -> Sum/1
  Product/1 -> Sum/2
  Product1/1 -> Sum/3
  Sum/1 -> Product2/1
  r_ABC/1 -> Product2/2
  Product2/1 -> Sum1/1
  m_sphere/1 -> Product3/1
  g/1 -> Product3/2
  Product3/1 -> Product4/2
  Xs/1 -> Product4/1
  Product4/1 -> Sum1/2
  Sum1/1 -> Divide/1
  Constant/1 -> Divide/2
  Divide/1 -> Product5/1
  Integrator/1 -> "d_theta "/1, Integrator1/1
  Integrator1/1 -> "theta "/1
  Product5/1 -> Integrator/1
  Constant1/1 -> Product5/2

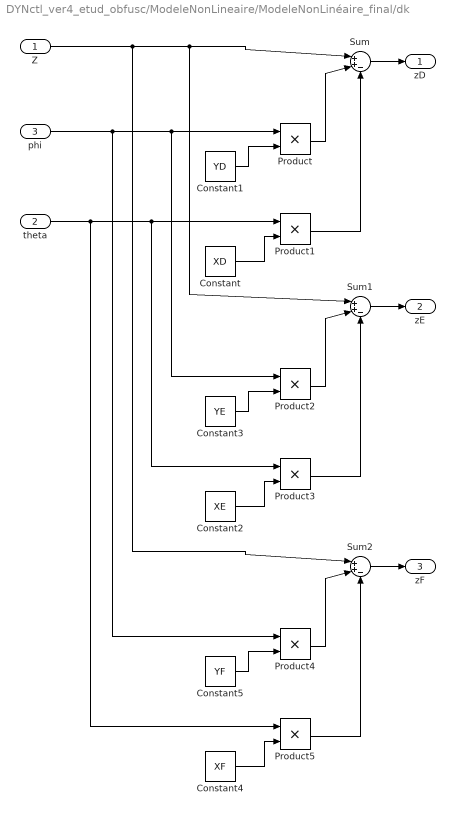
== system DYNctl_ver4_etud_obfusc/ModeleNonLineaire/ModeleNonLinéaire_final/dk ==
  Z : Inport
  theta : Inport  Port=2
  phi : Inport  Port=3
  Constant : Constant  Value=XD
  Constant1 : Constant  Value=YD
  Constant2 : Constant  Value=XE
  Constant3 : Constant  Value=YE
  Constant4 : Constant  Value=XF
  Constant5 : Constant  Value=YF
  Product{,1..5} (6 alike) : Product
  Sum : Sum  Inputs=|++-
  Sum1 : Sum  Inputs=|++-
  Sum2 : Sum  Inputs=|++-
  zD : Outport
  zE : Outport  Port=2
  zF : Outport  Port=3
  wires:
  Constant1/1 -> Product/2
  Product/1 -> Sum/2
  Constant/1 -> Product1/2
  Product1/1 -> Sum/3
  Sum/1 -> zD/1
  Constant3/1 -> Product2/2
  Product2/1 -> Sum1/2
  Constant2/1 -> Product3/2
  Product3/1 -> Sum1/3
  Sum1/1 -> zE/1
  phi/1 -> Product4/1, Product2/1, Product/1
  Constant5/1 -> Product4/2
  Product4/1 -> Sum2/2
  Z/1 -> Sum2/1, Sum1/1, Sum/1
  theta/1 -> Product5/1, Product3/1, Product1/1
  Constant4/1 -> Product5/2
  Product5/1 -> Sum2/3
  Sum2/1 -> zF/1
